simulink model "Cognata_Amp_Tobi"  (R2017a)
settings: Solver=ode45  StartTime=0.0  StopTime=inf  RelTol=1e-3
model workspace (MAT data in the model file):
  cfg_native : struct (value not decoded)
  en_add_channels = 1
  host_ip = 2130706433
  host_port = 50223
  local_ip = 2130706433
  local_port = 50224
  num_en_channels = 32
  num_samples = 1
  sample_rate = 250
  serial_number = 'NB-2015.10.93'
undefined symbols (not defined in the file or in its folder): currentCFG_Cognata_Amp_Tobi_UR, UR
libraries: simulink x1, TobiiEyeTrackerLib x1, robotlib x1, gtecHighspeedLib x1, gUSBamplib x1
settings Model: ModifiedByFormat=g.tec  Creator=g.tec medical engineering  LastModifiedBy=g.tec
settings DataIOCC: LimitDataPoints=on  SaveFormat=Array
settings OptimizationCC: BlockReduction=off  BooleanDataType=off  LifeSpan=inf
settings DebuggingCC: SaveWithParameterizedLinksMsg=none  UnderspecifiedInitializationDetection=Classic  MergeDetectMultiDrivingBlocksExec=none  SignalResolutionControl=TryResolveAllWithWarning  FrameProcessingCompatibilityMsg=none  SFUnexpectedBacktrackingDiag=warning  SFNoUnconditionalDefaultTransitionDiag=warning  SFExecutionAtInitializationDiag=none
settings HardwareCC: ProdBitPerPointer=32  ProdBitPerSizeT=32  ProdBitPerPtrDiffT=32  ProdLargestAtomicFloat=None  ProdIntDivRoundTo=Undefined  ProdEndianess=Unspecified  ProdWordSize=32  ProdHWDeviceType=32-bit Generic  TargetUnknown=on
settings ModelReferenceCC: PropagateSignalLabelsOutOfModel=off
settings GRTTargetCC: TargetLangStandard=C89/C90 (ANSI)  GeneratePreprocessorConditionals=Disable all
settings ConfigComp: CovMetricSettings=dw  CovHtmlReporting=on  CovSaveCumulativeToWorkspaceVar=on  CovSaveSingleToWorkspaceVar=on  CovExternalEMLEnable=off

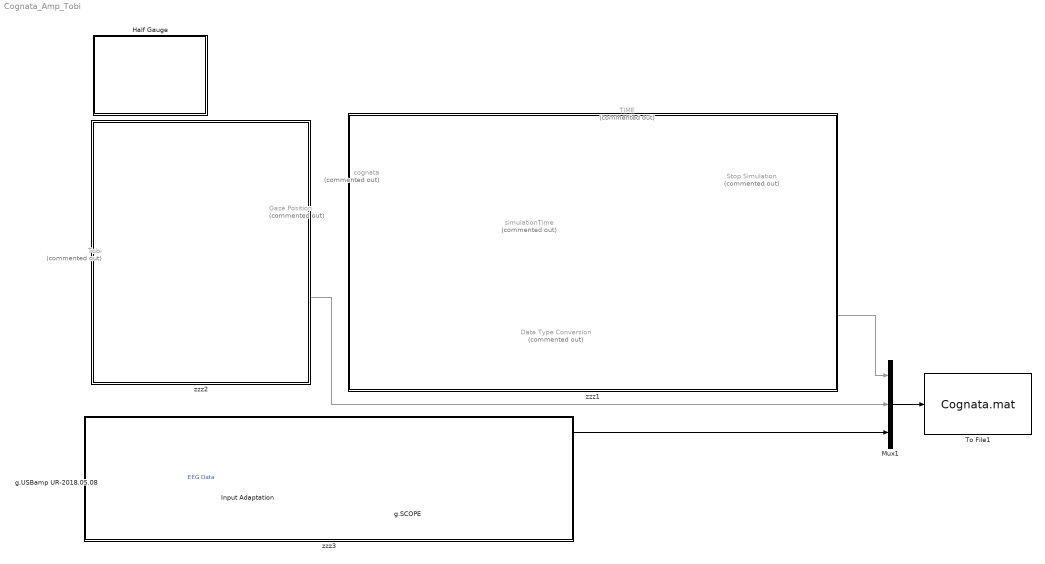
== system Cognata_Amp_Tobi ==
  Data Type Conversion : DataTypeConversion  Commented=on
  Gaze Position : Display  Commented=on
  Half Gauge : Subsystem  DialogController=hmiCreateDDGDialog  IsWebBlock=on  mask(MWDashboardBlock){webBlockId=e3860c53-3e23-4b65-a6ef-6d267d62b553, webBlockType=semicirculargauge, ShowInLibBrowser=on, ShowInitialText=on, HMISrcModelName=Cognata_Amp_Tobi}
      mask prompts: webBlockId "WebBlock Id"; webBlockType "WebBlock Type"; HMISrcModelName "Source Model"
      mask help: SimulinkHMI:dialogs:SemicircularGaugeDialogDesc
      mask Help: helpview([docroot '/mapfiles/simulink.map'], 'hmi_half_gauge')
      mask Display:
      | if strcmp(get_param(bdroot(gcb),'BlockDiagramType'), 'library')
      |     image([(matlabroot) '/toolbox/simulink/hmi/icons/SemicircularGauge.png']);
      | end
  Input Adaptation : Subsystem
  Mux1 : Mux  Inputs=3
  Stop Simulation : Stop  Commented=on
  TIME : simulink/Logic and Bit Operations/Compare To Constant  Commented=on  relop=>=  const=15  OutDataTypeStr=boolean
  To File1 : ToFile  Filename=Cognata.mat  MatrixName=data  SampleTime=0.03
  Tobi : Subsystem  Commented=on
  cognata : Subsystem  Commented=on
  g.SCOPE : gtecHighspeedLib/g.SCOPE
      settings: SourceProductName=g.HIsys Library
  g.USBamp UR-2018.05.08 : gUSBamplib/g.USBamp  cfg=currentCFG_Cognata_Amp_Tobi_UR-2018.05.08.cfg  snr=UR-2018.05.08
      settings: SourceProductName=g.USBamp
  simulationTime : Display  Commented=on
  zzz1 : Subsystem  TreatAsAtomicUnit=on
      settings: OpenFcn=% no-op
      mask Display: disp('')
  zzz2 : Subsystem  TreatAsAtomicUnit=on
      settings: OpenFcn=% no-op
      mask Display: disp('')
  zzz3 : Subsystem  TreatAsAtomicUnit=on
      settings: OpenFcn=% no-op
      mask Display: disp('')
  wires:
  g.USBamp UR-2018.05.08/1 -> Input Adaptation/1(In)  "EEG Data"
  TIME/1 -> Stop Simulation/1
  cognata/1(SimulationTime) -> TIME/1, Data Type Conversion/1, simulationTime/1
  Mux1/1 -> To File1/1
  Tobi/1(Gaze Pos) -> Gaze Position/1
  Tobi/2(Sum) -> Mux1/2
  Input Adaptation/1(Out) -> Mux1/3, g.SCOPE/1
  Data Type Conversion/1 -> Mux1/1

== system Cognata_Amp_Tobi/Half Gauge ==

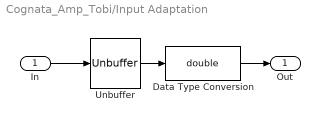
== system Cognata_Amp_Tobi/Input Adaptation ==
  In : Inport
  Data Type Conversion : DataTypeConversion  OutDataTypeStr=double
  Unbuffer : Unbuffer
  Out : Outport
  wires:
  In/1 -> Unbuffer/1
  Unbuffer/1 -> Data Type Conversion/1
  Data Type Conversion/1 -> Out/1

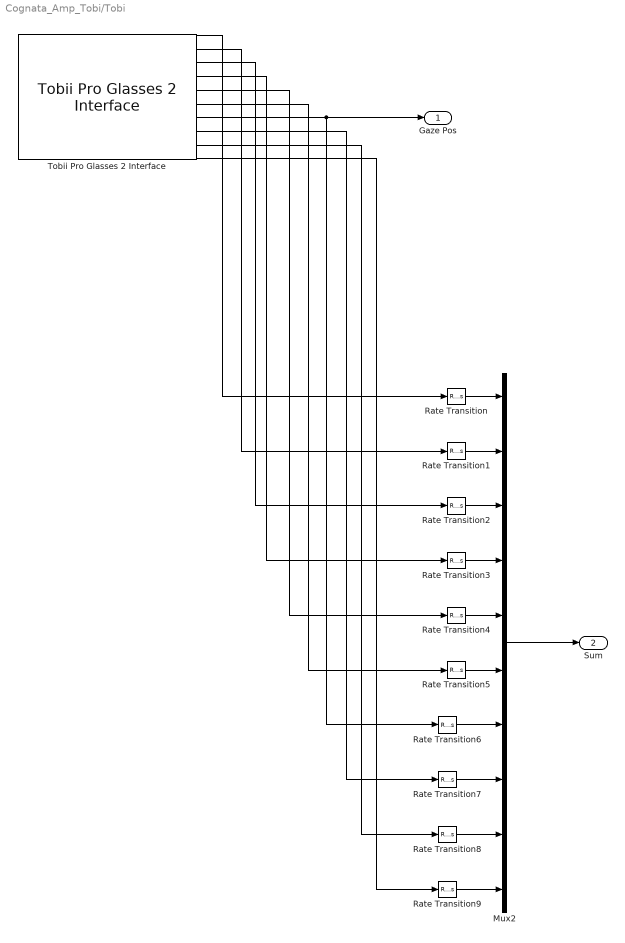
== system Cognata_Amp_Tobi/Tobi ==
  Mux2 : Mux  Inputs=10
  Rate Transition{,1..9} (10 alike) : RateTransition  Deterministic=off  OutPortSampleTimeOpt=Inherit
  Tobii Pro Glasses 2 Interface : TobiiEyeTrackerLib/Tobii Pro Glasses 2 Interface  Key=0  pc_right=off  pc_left=off  pd_right=off  pd_left=off  gd_right=off  gd_left=off  gp=on  gp3=off  gy=off  ac=off
      settings: SourceProductName=g.EYEtracking Interface (Tobii Pro Glasses 2)
  Gaze Pos : Outport
  Sum : Outport  Port=2
  wires:
  Rate Transition1/1 -> Mux2/2
  Rate Transition9/1 -> Mux2/10
  Rate Transition6/1 -> Mux2/7
  Rate Transition7/1 -> Mux2/8
  Rate Transition8/1 -> Mux2/9
  Rate Transition/1 -> Mux2/1
  Rate Transition3/1 -> Mux2/4
  Rate Transition5/1 -> Mux2/6
  Rate Transition4/1 -> Mux2/5
  Mux2/1 -> Sum/1
  Rate Transition2/1 -> Mux2/3
  Tobii Pro Glasses 2 Interface/8 -> Rate Transition7/1
  Tobii Pro Glasses 2 Interface/2 -> Rate Transition1/1
  Tobii Pro Glasses 2 Interface/10 -> Rate Transition9/1
  Tobii Pro Glasses 2 Interface/9 -> Rate Transition8/1
  Tobii Pro Glasses 2 Interface/4 -> Rate Transition3/1
  Tobii Pro Glasses 2 Interface/7 -> Gaze Pos/1, Rate Transition6/1
  Tobii Pro Glasses 2 Interface/6 -> Rate Transition5/1
  Tobii Pro Glasses 2 Interface/1 -> Rate Transition/1
  Tobii Pro Glasses 2 Interface/3 -> Rate Transition2/1
  Tobii Pro Glasses 2 Interface/5 -> Rate Transition4/1

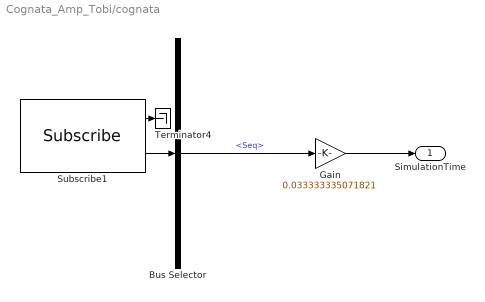
== system Cognata_Amp_Tobi/cognata ==
  Bus Selector : BusSelector  OutputSignals=Header.Seq
  Gain : Gain  Gain=0.033333335071821
  Subscribe1 : robotlib/Subscribe  SourceLibraryInfo=This block requires Robotics System Toolbox  topicSource=Select from ROS network  topic=/cognataSDK/GPS/info  messageType=sensor_msgs/NavSatFix  sampleTime=-1  messageQueueLength=10
      settings: SourceProductBaseCode=RO
  Terminator4 : Terminator
  SimulationTime : Outport
  wires:
  Bus Selector/1 -> Gain/1  "<Seq>"
  Subscribe1/2 -> Bus Selector/1
  Gain/1 -> SimulationTime/1
  Subscribe1/1 -> Terminator4/1

== system Cognata_Amp_Tobi/zzz1 ==

== system Cognata_Amp_Tobi/zzz2 ==

== system Cognata_Amp_Tobi/zzz3 ==
